simulink model "Ex10_2_2_ExportingToWorkspace"  (R2023a)
settings: Solver=VariableStepAuto  StartTime=0.0  StopTime=13.0  RelTol=1e-3
settings Model: Creator=Norb  LastModifiedBy=Norb

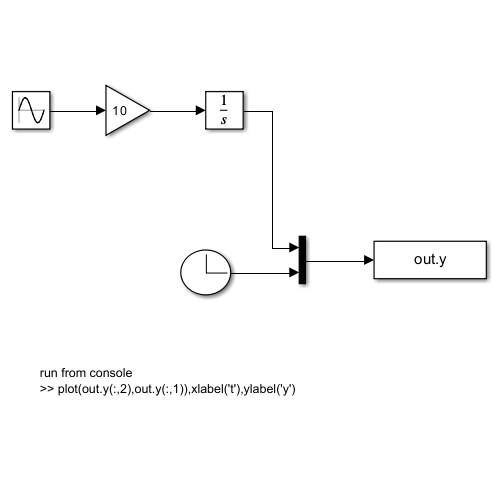
[thumbnail: Simulink's stored preview of the top-level diagram]
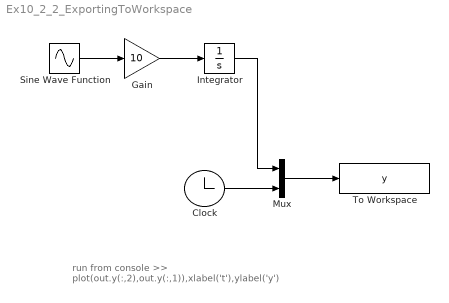
== system Ex10_2_2_ExportingToWorkspace ==
  note: run from console
      | >> plot(out.y(:,2),out.y(:,1)),xlabel('t'),ylabel('y')
  Clock : Clock
  Gain : Gain  Gain=10
  Integrator : Integrator
  Mux : Mux  Inputs=2
  Sine Wave Function : Sin  SampleTime=0
  To Workspace : ToWorkspace  VariableName=y  SampleTime=-1
  wires:
  Sine Wave Function/1 -> Gain/1
  Gain/1 -> Integrator/1
  Integrator/1 -> Mux/1
  Clock/1 -> Mux/2
  Mux/1 -> To Workspace/1
